simulink model "OpAmpLab_SolnPart2"  (R2021b)
settings: Solver=VariableStepAuto  StartTime=0.0  StopTime=inf  MaxStep=1e-5  RelTol=1e-3
libraries: fl_lib x13, nesl_utility x3
settings Model: PacingRate=0.010000  Creator=Work  LastModifiedBy=Work

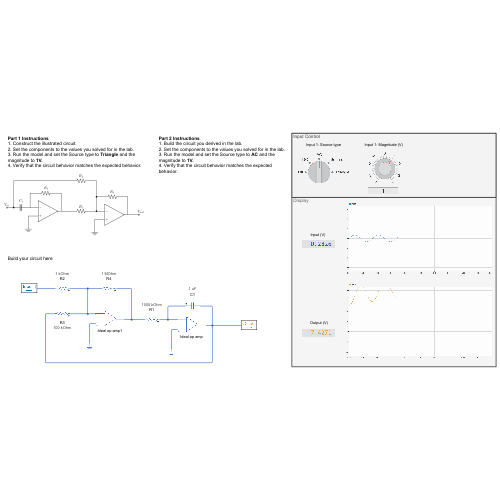
[thumbnail: Simulink's stored preview of the top-level diagram]
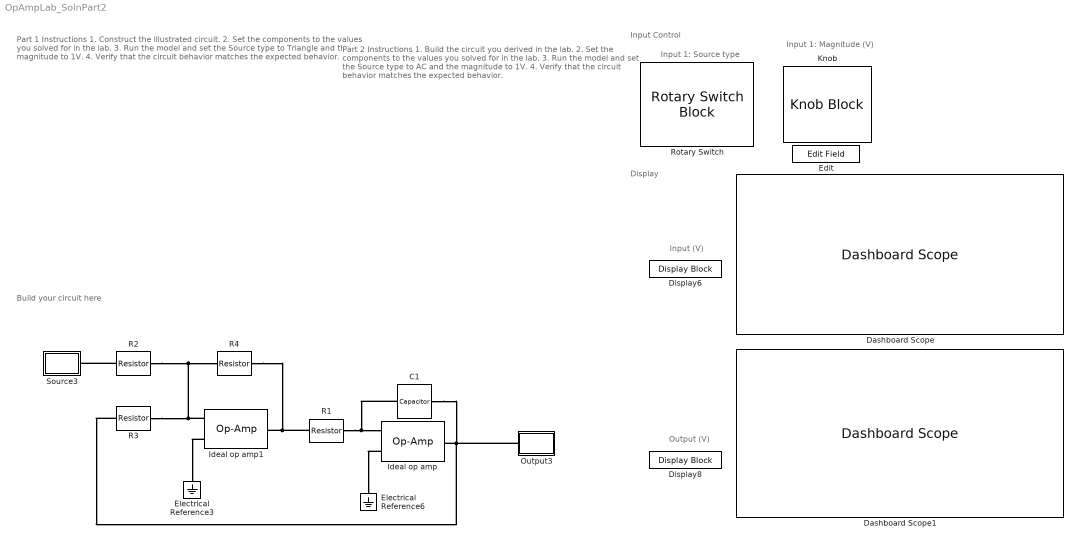
== system OpAmpLab_SolnPart2 ==
  note: Build your circuit here
  note: Input 1: Magnitude (V)
  note: Input 1: Source type
  note: Input Control
  note: Display
  note: Input (V)
  note: Output (V)
  note: Part 1 Instructions
      | 1. Construct the illustrated circuit.
      | 2. Set the components to the values you solved for in the lab.
      | 3. Run the model and set the Source type to Triangle and the magnitude to 1V.
      | 4. Verify that the circuit behavior matches the expected behavior.
  note: Part 2 Instructions
      | 1. Build the circuit you derived in the lab.
      | 2. Set the components to the values you solved for in the lab.
      | 3. Run the model and set the Source type to AC and the magnitude to 1V.
      | 4. Verify that the circuit behavior matches the expected behavior.
  C1 : fl_lib/Electrical/Electrical Elements/Capacitor  c=1 uF  r=1e-6 Ohm  g=0 1/Ohm  i_specify=off  i_priority=None  i=0 A  i_nominal_specify=off  i_nominal_unit=A  i_nominal_value=1  v_specify=off  v_priority=None  v=0 V  v_nominal_specify=off  v_nominal_unit=V  v_nominal_value=1  vc_specify=off  vc_priority=High  vc=0 V  vc_nominal_specify=off  vc_nominal_unit=V  vc_nominal_value=1
      settings: AttributesFormatString=%<c> %<c_unit>
  Dashboard Scope : DashboardScope  TimeSpan=0.10000000000000001  Ymin=-10  Ymax=10  ScaleAtStop=off
  Dashboard Scope1 : DashboardScope  TimeSpan=0.10000000000000001  Ymin=-10  Ymax=10  ScaleAtStop=off
  Display6 : DisplayBlock  LabelPosition=Hide  Format=Custom  Alignment=Right  Transparency=1  FormatString=%0.4f
  Display8 : DisplayBlock  LabelPosition=Hide  Format=Custom  Alignment=Right  Transparency=1  FormatString=%0.4f
  Edit : EditField  LabelPosition=Hide  ShowInitialText=on  Alignment=Center
  Electrical Reference3 : fl_lib/Electrical/Electrical Elements/Electrical Reference
  Electrical Reference6 : fl_lib/Electrical/Electrical Elements/Electrical Reference
  Ideal op amp : fl_lib/Electrical/Electrical Elements/Op-Amp  outI_specify=off  outI_priority=None  outI=0 A  outI_nominal_specify=off  outI_nominal_unit=A  outI_nominal_value=1
  Ideal op amp1 : fl_lib/Electrical/Electrical Elements/Op-Amp  outI_specify=off  outI_priority=None  outI=0 A  outI_nominal_specify=off  outI_nominal_unit=A  outI_nominal_value=1
  Knob : KnobBlock  LabelPosition=Hide  ScaleMin=-4  ScaleMax=4  TickInterval=1
  Output3 : Subsystem
      mask Display: image("output.png")
  R1 : fl_lib/Electrical/Electrical Elements/Resistor  R=1000 kOhm  i_specify=off  i_priority=None  i=0 A  i_nominal_specify=off  i_nominal_unit=A  i_nominal_value=1  v_specify=off  v_priority=None  v=0 V  v_nominal_specify=off  v_nominal_unit=V  v_nominal_value=1
      settings: AttributesFormatString=%<R> %<R_unit>
  R2 : fl_lib/Electrical/Electrical Elements/Resistor  R=1 kOhm  i_specify=off  i_priority=None  i=0 A  i_nominal_specify=off  i_nominal_unit=A  i_nominal_value=1  v_specify=off  v_priority=None  v=0 V  v_nominal_specify=off  v_nominal_unit=V  v_nominal_value=1
      settings: AttributesFormatString=%<R> %<R_unit>
  R3 : fl_lib/Electrical/Electrical Elements/Resistor  R=100 kOhm  i_specify=off  i_priority=None  i=0 A  i_nominal_specify=off  i_nominal_unit=A  i_nominal_value=1  v_specify=off  v_priority=None  v=0 V  v_nominal_specify=off  v_nominal_unit=V  v_nominal_value=1
      settings: AttributesFormatString=%<R> %<R_unit>
  R4 : fl_lib/Electrical/Electrical Elements/Resistor  R=1 MOhm  i_specify=off  i_priority=None  i=0 A  i_nominal_specify=off  i_nominal_unit=A  i_nominal_value=1  v_specify=off  v_priority=None  v=0 V  v_nominal_specify=off  v_nominal_unit=V  v_nominal_value=1
      settings: AttributesFormatString=%<R> %<R_unit>
  Rotary Switch : RotarySwitchBlock  LabelPosition=Hide
      settings: Values={{'Off', 'DC', 'AC', 'Square', 'Triangle'}, [0 1 2 3 4]}
  Source3 : Subsystem
      mask Display: image("input1.png")
  connections:
  Ideal op amp1/LConn2 -- R3/LConn1 -- R2/LConn1 -- R4/RConn1
  R4/LConn1 -- Ideal op amp1/RConn1 -- R1/RConn1
  Ideal op amp1/LConn1 -- Electrical Reference3/LConn1
  Ideal op amp/LConn1 -- Electrical Reference6/LConn1
  R1/LConn1 -- C1/LConn1 -- Ideal op amp/LConn2
  C1/RConn1 -- R3/RConn1 -- Output3/LConn1 -- Ideal op amp/RConn1
  R2/RConn1 -- Source3/RConn1

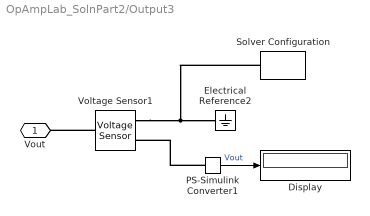
== system OpAmpLab_SolnPart2/Output3 ==
  Display : Display
  Electrical Reference2 : fl_lib/Electrical/Electrical Elements/Electrical Reference
  PS-Simulink Converter1 : nesl_utility/PS-Simulink Converter  PhysicalDomain=network_engine_domain  SubClassName=ps_output  LeftPortType=input  RightPortType=output  PseudoPeriodic=off  Frequencies=[]  Unit=inherit  AffineConversion=off
      settings: SourceProductBaseCode=PW,SS
  Solver Configuration : nesl_utility/Solver Configuration  PhysicalDomain=network_engine_domain  SubClassName=solver  LeftPortType=input  RightPortType=generic  Tones=[]  Harmonics=[]  SimulateNoise=off  Profile=off  UseLocalSampling=off  EnableSwitchedLinearOptims=on  FrequencyDomain=off  UseCCode=off  RelTol=0.001  AbsTol=1e-06  MinStep=1e-09  ToWorkspace=off  RevertToSquareIcSolve=off  NumHomotopyIterations=100  PhasorMode=off  PhasorModeNumHarmonics=1  DoDC=off  ResidualTolerance=1e-09  UseLocalSolver=off  LocalSolverChoice=NE_BACKWARD_EULER_ADVANCER  LocalSolverSampleTime=0.001  DoFixedCost=off  MaxNonlinIter=3  MaxModeIter=2  ComputeImpulses=off  ImpulseIterations=2  LinearAlgebra=auto  EquationFormulation=NE_TIME_EF  DelaysMemoryBudget=1024  AutomaticFiltering=on  FilteringTimeConstant=0.001  PartitionStorageMethod=AS_NEEDED  PartitionMemoryBudget=1024  PartitionMethod=ROBUST
      settings: SourceProductBaseCode=PW,SS
  Voltage Sensor1 : fl_lib/Electrical/Electrical Sensors/Voltage Sensor
  Vout : PMIOPort  Side=Left
  wires:
  PS-Simulink Converter1/1 -> Display/1  "Vout"
  connections:
  Voltage Sensor1/LConn1 -- Vout/RConn1
  Voltage Sensor1/RConn2 -- Solver Configuration/RConn1 -- Electrical Reference2/LConn1
  PS-Simulink Converter1/LConn1 -- Voltage Sensor1/RConn1

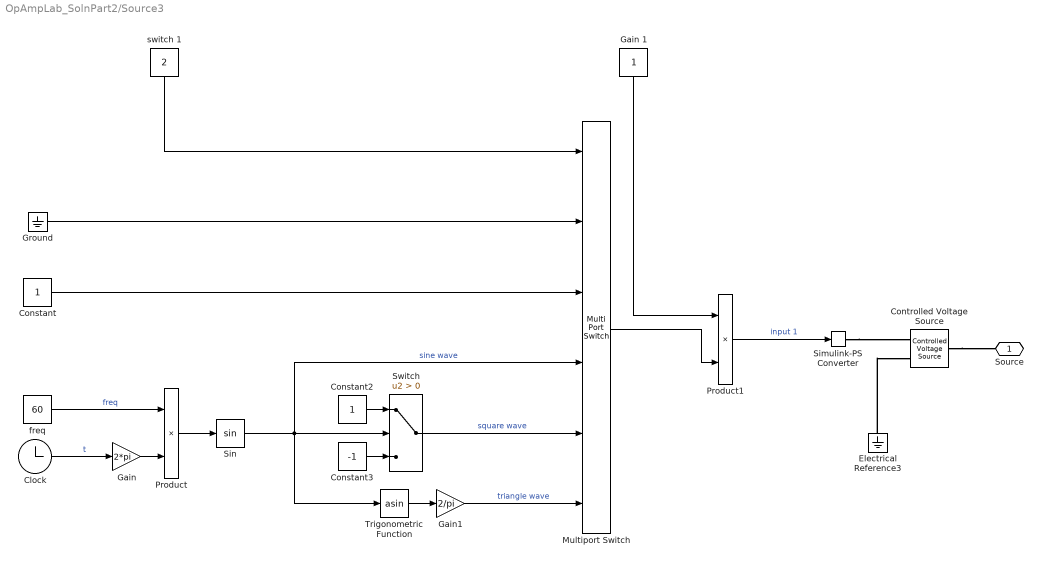
== system OpAmpLab_SolnPart2/Source3 ==
  Clock : Clock
  Constant : Constant
  Constant2 : Constant  SampleTime=0
  Constant3 : Constant  Value=-1  SampleTime=0
  Controlled Voltage Source : fl_lib/Electrical/Electrical Sources/Controlled Voltage Source
  Electrical Reference3 : fl_lib/Electrical/Electrical Elements/Electrical Reference
  Gain : Gain  Gain=2*pi
  Gain 1 : Constant
  Gain1 : Gain  Gain=2/pi
  Ground : Ground
  Multiport Switch : MultiPortSwitch  DataPortOrder=Zero-based contiguous  Inputs=5  zeroidx=on
  Product : Product
  Product1 : Product
  Simulink-PS Converter : nesl_utility/Simulink-PS Converter  PhysicalDomain=network_engine_domain  SubClassName=ps_input  LeftPortType=input  RightPortType=output  PseudoPeriodic=off  Frequencies=[]  NoiseDistribution=none  NoiseParameters=[]  Unit=1  AffineConversion=off  FilteringAndDerivatives=provide  SimscapeFilterOrder=1  InputFilterTimeConstant=0.001  UdotUserProvided=0
      settings: SourceProductBaseCode=PW,SS
  Sin : Trigonometry
  Switch : Switch  Criteria=u2 > Threshold
  Trigonometric Function : Trigonometry  Operator=asin
  freq : Constant  Value=60  SampleTime=0
  switch 1 : Constant  Value=2
  Source : PMIOPort  Side=Right
  wires:
  Multiport Switch/1 -> Product1/2
  Product1/1 -> Simulink-PS Converter/1  "input 1"
  Product/1 -> Sin/1
  Gain 1/1 -> Product1/1
  Constant3/1 -> Switch/3
  Constant/1 -> Multiport Switch/3
  Clock/1 -> Gain/1  "t"
  freq/1 -> Product/1  "freq"
  Switch/1 -> Multiport Switch/5  "square wave"
  Trigonometric Function/1 -> Gain1/1
  Gain/1 -> Product/2
  Constant2/1 -> Switch/1
  Sin/1 -> Multiport Switch/4, Trigonometric Function/1, Switch/2  "sine wave"
  switch 1/1 -> Multiport Switch/1
  Gain1/1 -> Multiport Switch/6  "triangle wave"
  Ground/1 -> Multiport Switch/2
  connections:
  Electrical Reference3/LConn1 -- Controlled Voltage Source/RConn2
  Controlled Voltage Source/LConn1 -- Source/RConn1
  Simulink-PS Converter/RConn1 -- Controlled Voltage Source/RConn1
